simulink model "assignment2"  (R2020b)
settings: Solver=VariableStepAuto  StartTime=0.0  StopTime=10.0  RelTol=1e-3
settings Model: Creator=Sudhanshu  LastModifiedBy=Sudhanshu

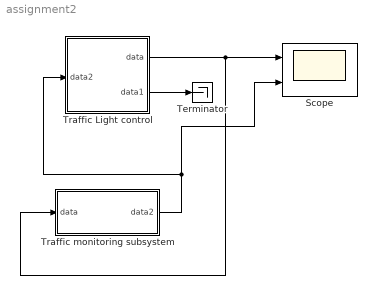
== system assignment2 ==
  Scope : Scope  NumInputPorts=2
  Terminator : Terminator
  Traffic Light control : Stateflow chart  TreatAsAtomicUnit=on
  Traffic monitoring subsystem : Subsystem
  wires:
  Traffic Light control/1(data) -> Traffic monitoring subsystem/1(data), Scope/1
  Traffic Light control/2(data1) -> Terminator/1
  Traffic monitoring subsystem/1(data2) -> Traffic Light control/1(data2), Scope/2

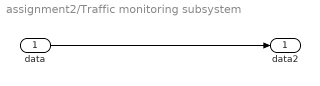
== system assignment2/Traffic monitoring subsystem ==
  data : Inport
  data2 : Outport
  wires:
  data/1 -> data2/1

== stateflow chart assignment2/Traffic Light control ==
  settings: stateMachineType=MOORE_MACHINE  initializeOutput=1
  state Stop
    signal1 = RED;
    signal2 = GREEN;
  state Stop_traffic
    signal1 = RED;
    signal2 = GREEN;
  state Stop_move
    signal1 = RED;
    signal2 = YELLOW;
  state Move
    signal1 = GREEN;
    signal2 = RED;
  state Move_stop
    signal1 = YELLOW;
    signal2 = RED;
  (default) -> Stop
  Stop -> Stop_traffic : after(20,tick)
  Stop_traffic -> Stop_move : [sens]
  Move_stop -> Stop : after (3,tick)
  Stop_move -> Move : after(3,tick)
  Move -> Move_stop : after(10,tick)
  data: data output double; data1 output double; data2 input double
